simulink model "minimal_task"  (Simulink 3.0)
libraries: mathlib x3, speclib x1, arclib x1

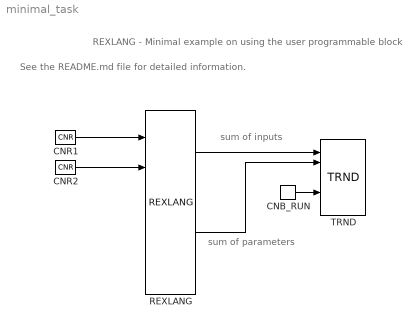
== system minimal_task ==
  note: sum of inputs
  note: sum of parameters
  note: REXLANG - Minimal example on using the user programmable block
  note: See the README.md file for detailed information.
  CNB_RUN : mathlib/CNB  YCN=on
  CNR1 : mathlib/CNR  SystemSampleTime=-1  ycn=3.7
  CNR2 : mathlib/CNR  SystemSampleTime=-1  ycn=4.3
  REXLANG : speclib/REXLANG  strs=0  SystemSampleTime=-1  tab_matlab=BASIC  srcname=minimal_rexlang.c  srctype=1: C-like  stack=0  debug=1: No check  p0=2.6  p1=8.9  p2=0  p3=0  p4=0  p5=0  p6=0  p7=0  p8=0  p9=0  p10=0  p11=0  p12=0  p13=0  p14=0  p15=0
  TRND : arclib/TRND  n=2  l=1000  btype=8: Double  ptype1=1: Store  ptype2=1: Store  ptype3=1: Store  ptype4=1: Store  pfac=1  afac=0  arc=0  id=1  Title=Trend Title  timesrc=1
  wires:
  CNB_RUN/1 -> TRND/5
  CNR1/1 -> REXLANG/3
  CNR2/1 -> REXLANG/6
  REXLANG/4 -> TRND/1
  REXLANG/12 -> TRND/2
